simulink model "Sim_Riementrieb"  (R2015b)
settings: Solver=ode45  StartTime=0.0  StopTime=12  MaxStep=1e-3  RelTol=1e-7  AbsTol=1e-7
InitFcn:
  | set_parameter
undefined symbols (not defined in the file or in its folder): parRegid, parRegomegam, parSys
libraries: cstblocks x2
settings Model: Creator=wke  LastModifiedBy=jens
settings SolverCC: ShapePreserveControl=EnableAll
settings DataIOCC: SaveFormat=Array  SignalLoggingSaveFormat=ModelDataLogs
settings OptimizationCC: ExpressionDepthLimit=2147483647
settings DebuggingCC: UnderspecifiedInitializationDetection=Classic  MergeDetectMultiDrivingBlocksExec=none  SolverPrmCheckMsg=warning  FcnCallInpInsideContextMsg=UseLocalSettings  StateNameClashWarn=warning
settings HardwareCC: ProdBitPerPointer=32  ProdLargestAtomicFloat=None  ProdIntDivRoundTo=Undefined  ProdEndianess=Unspecified  ProdWordSize=32  ProdHWDeviceType=32-bit Generic
settings SFSimCC: SimParseCustomCode=off
settings GRTTargetCC: GeneratePreprocessorConditionals=Disable all  CombineOutputUpdateFcns=off  GRTInterface=on
settings ConfigComp: CovModelRefEnable=Off

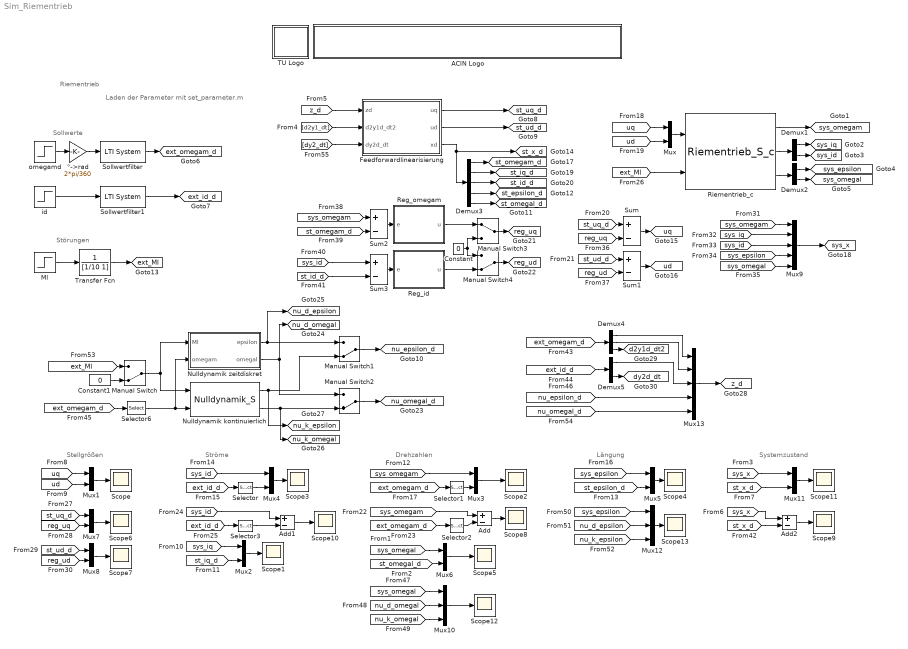
== system Sim_Riementrieb ==
  note: Riementrieb
  note: Laden der Parameter mit set_parameter.m
  note: Sollwerte
  note: Stellgrößen
  note: Ströme
  note: Drehzahlen
  note: Längung
  note: Störungen
  note: Systemzustand
  ACIN Logo : Subsystem
      mask init:
      | s = get_param(gcb,'UserData');
      mask Display:
      | image(s.logo,[0 0 439 45]);
      | %axis image
  Add : Sum  Inputs=+-
  Add1 : Sum  Inputs=+-
  Add2 : Sum  Inputs=+-
  Constant : Constant  Value=0
  Constant1 : Constant  Value=0
  Demux1 : Demux  Outputs=2
  Demux2 : Demux  Outputs=2
  Demux3 : Demux  Outputs=5
  Demux4 : Demux  Outputs=3
  Demux5 : Demux  Outputs=2
  Feedforwardlinearisierung : MATLAB Function  TreatAsAtomicUnit=on
  Manual Switch{,1..2,4} (4 alike) : ManualSwitch  CurrentSetting=0
  Manual Switch3 : ManualSwitch
  Ml : Step  Time=8  After=0.1  SampleTime=0
  Mux{,1..8,11} (10 alike) : Mux  Inputs=2
  Mux10 : Mux  Inputs=3
  Mux12 : Mux  Inputs=3
  Mux13 : Mux  Inputs=5
  Mux9 : Mux  Inputs=5
  Nulldynamik kontinuierlich : M-S-Function  FunctionName=Nulldynamik_S  Parameters=parSys
  Nulldynamik zeitdiskret : MATLAB Function  TreatAsAtomicUnit=on
  Reg_id : MATLAB Function  TreatAsAtomicUnit=on
  Reg_omegam : MATLAB Function  TreatAsAtomicUnit=on
  Riementrieb_c : S-Function  FunctionName=Riementrieb_S_c  Parameters=parSys  SFunctionDeploymentMode=off  EnableBusSupport=off
      mask Display:
      | port_label('input',1,'uq,ud');
      | port_label('input',2,'Ml');
      | port_label('output',1,'omegam');
      | port_label('output',2,'iq,id');
      | port_label('output',3,'epsilon,omegal');
  Scope{,1..13} (14 alike) : Scope
  Selector : Selector  InputPortWidth=2  IndexOptions=Index vector (dialog)  Indices=[1]  OutputSizes=1
  Selector1 : Selector  InputPortWidth=3  IndexOptions=Index vector (dialog)  Indices=[1]  OutputSizes=1
  Selector2 : Selector  InputPortWidth=3  IndexOptions=Index vector (dialog)  Indices=[1]  OutputSizes=1
  Selector3 : Selector  InputPortWidth=2  IndexOptions=Index vector (dialog)  Indices=[1]  OutputSizes=1
  Selector6 : Selector  InputPortWidth=3  IndexOptions=Index vector (dialog)  Indices=[1]  OutputSizes=1
  Sollwertfilter : cstblocks/LTI System  sys=parReg.ssSF  IC=[]
  Sollwertfilter1 : cstblocks/LTI System  sys=parReg.ssSFi  IC=[]
  Sum{,1..3} (4 alike) : Sum  Inputs=+-
  TU Logo : Subsystem
      mask init:
      | s = get_param(gcb,'UserData');
      mask Display: image(s.logo,[0 0 45 45]);
  Transfer Fcn : TransferFcn  Denominator=[1/10 1]
  id : Step  After=0.1  SampleTime=0
  omegamd : Step  Time=4  After=1000/60*360  SampleTime=0
  °->rad : Gain  Gain=2*pi/360
  tag scope: d2y1d_dt2=global, dy2d_dt=global, ext_Ml=global, ext_id_d=global, ext_omegam_d=global, nu_d_epsilon=global, nu_d_omegal=global, nu_epsilon_d=global, nu_k_epsilon=global, nu_k_omegal=global, nu_omegal_d=global, reg_ud=global, reg_uq=global, st_epsilon_d=global, st_id_d=global, st_iq_d=global, st_omegal_d=global, st_omegam_d=global, st_ud_d=global, st_uq_d=global, st_x_d=global, sys_epsilon=global, sys_id=global, sys_iq=global, sys_omegal=global, sys_omegam=global, sys_x=global, ud=global, uq=global, z_d=global
  wires:
  Mux/1 -> Riementrieb_c/1
  °->rad/1 -> Sollwertfilter/1
  Sollwertfilter/1 -> [ext_omegam_d]
  Demux1/1 -> [sys_iq]
  Demux1/2 -> [sys_id]
  Demux2/1 -> [sys_epsilon]
  Demux2/2 -> [sys_omegal]
  Sollwertfilter1/1 -> [ext_id_d]
  id/1 -> Sollwertfilter1/1
  [uq] -> Mux1/1
  [ud] -> Mux1/2
  Mux1/1 -> Scope/1
  [sys_iq] -> Mux2/1
  [st_iq_d] -> Mux2/2
  Mux2/1 -> Scope1/1
  [sys_omegam] -> Mux3/1
  Mux3/1 -> Scope2/1
  [sys_id] -> Mux4/1
  [ext_id_d] -> Selector/1
  Mux4/1 -> Scope3/1
  [sys_epsilon] -> Mux5/1
  Mux5/1 -> Scope4/1
  [sys_omegal] -> Mux6/1
  Mux6/1 -> Scope5/1
  [ext_omegam_d] -> Selector1/1
  Selector1/1 -> Mux3/2
  Selector/1 -> Mux4/2
  [st_epsilon_d] -> Mux5/2
  [st_omegal_d] -> Mux6/2
  Add/1 -> Scope8/1
  [sys_omegam] -> Add/1
  [ext_omegam_d] -> Selector2/1
  Selector2/1 -> Add/2
  Add1/1 -> Scope10/1
  [sys_id] -> Add1/1
  [ext_id_d] -> Selector3/1
  Selector3/1 -> Add1/2
  Ml/1 -> Transfer Fcn/1
  omegamd/1 -> °->rad/1
  Transfer Fcn/1 -> [ext_Ml]
  [ext_Ml] -> Riementrieb_c/2
  [st_uq_d] -> Mux7/1
  [reg_uq] -> Mux7/2
  Mux7/1 -> Scope6/1
  [st_ud_d] -> Mux8/1
  [reg_ud] -> Mux8/2
  Mux8/1 -> Scope7/1
  Riementrieb_c/2 -> Demux1/1
  Riementrieb_c/3 -> Demux2/1
  Riementrieb_c/1 -> [sys_omegam]
  [sys_omegam] -> Mux9/1
  [sys_iq] -> Mux9/2
  [sys_id] -> Mux9/3
  [sys_epsilon] -> Mux9/4
  [sys_omegal] -> Mux9/5
  Mux9/1 -> [sys_x]
  Mux11/1 -> Scope11/1
  [sys_x] -> Mux11/1
  [st_x_d] -> Mux11/2
  [uq] -> Mux/1
  [ud] -> Mux/2
  Demux3/4 -> [st_epsilon_d]
  Demux3/5 -> [st_omegal_d]
  Demux3/1 -> [st_omegam_d]
  Demux3/2 -> [st_iq_d]
  Demux3/3 -> [st_id_d]
  Add2/1 -> Scope9/1
  [sys_x] -> Add2/1
  [st_x_d] -> Add2/2
  [z_d] -> Feedforwardlinearisierung/1(zd)
  Feedforwardlinearisierung/1(uq) -> [st_uq_d]
  Feedforwardlinearisierung/2(ud) -> [st_ud_d]
  Feedforwardlinearisierung/3(xd) -> Demux3/1, [st_x_d]
  Nulldynamik zeitdiskret/1(epsilon) -> [nu_d_epsilon], Manual Switch1/1
  Nulldynamik zeitdiskret/2(omegal) -> [nu_d_omegal], Manual Switch2/1
  Nulldynamik kontinuierlich/1 -> [nu_k_epsilon], Manual Switch1/2
  Nulldynamik kontinuierlich/2 -> [nu_k_omegal], Manual Switch2/2
  [sys_omegal] -> Mux10/1
  [nu_d_omegal] -> Mux10/2
  [nu_k_omegal] -> Mux10/3
  Mux10/1 -> Scope12/1
  [ext_omegam_d] -> Selector6/1
  Selector6/1 -> Nulldynamik zeitdiskret/2(omegam), Nulldynamik kontinuierlich/2
  [sys_epsilon] -> Mux12/1
  [nu_d_epsilon] -> Mux12/2
  [nu_k_epsilon] -> Mux12/3
  Mux12/1 -> Scope13/1
  [ext_Ml] -> Manual Switch/1
  Constant1/1 -> Manual Switch/2
  Manual Switch/1 -> Nulldynamik zeitdiskret/1(Ml), Nulldynamik kontinuierlich/1
  Manual Switch1/1 -> [nu_epsilon_d]
  Manual Switch2/1 -> [nu_omegal_d]
  Mux13/1 -> [z_d]
  [ext_omegam_d] -> Demux4/1
  Demux4/1 -> Mux13/1
  Demux4/2 -> Mux13/2
  [ext_id_d] -> Demux5/1
  Demux5/1 -> Mux13/3
  [nu_omegal_d] -> Mux13/5
  [nu_epsilon_d] -> Mux13/4
  Demux4/3 -> [d2y1d_dt2]
  Demux5/2 -> [dy2d_dt]
  [d2y1_dt] -> Feedforwardlinearisierung/2(d2y1d_dt2)
  [dy2_dt] -> Feedforwardlinearisierung/3(dy2d_dt)
  Sum/1 -> [uq]
  [reg_uq] -> Sum/2
  [st_uq_d] -> Sum/1
  Sum1/1 -> [ud]
  [st_ud_d] -> Sum1/1
  [reg_ud] -> Sum1/2
  Manual Switch3/1 -> [reg_uq]
  Manual Switch4/1 -> [reg_ud]
  Constant/1 -> Manual Switch3/2, Manual Switch4/1
  Reg_id/1(u) -> Manual Switch4/2
  Reg_omegam/1(u) -> Manual Switch3/1
  [sys_omegam] -> Sum2/1
  [st_omegam_d] -> Sum2/2
  Sum3/1 -> Reg_id/1(e)
  Sum2/1 -> Reg_omegam/1(e)
  [sys_id] -> Sum3/1
  [st_id_d] -> Sum3/2

== system Sim_Riementrieb/ACIN Logo ==

== system Sim_Riementrieb/TU Logo ==

== matlab function Sim_Riementrieb/Nulldynamik zeitdiskret ==
  settings: updateMethod=DISCRETE  sampleTime=parSys.TsID
  data: Ml input; omegam input; epsilon output; parSys parameter; omegal output
function [epsilon, omegal] = fcn(Ml,omegam,parSys)
%#codegen

persistent etakm1;
persistent ukm1;

if isempty(etakm1) || isempty(ukm1)
    etakm1  = [parSys.eta_1_0 parSys.eta_2_0];
    ukm1    = [Ml omegam];
    epsilon = etakm1(1);
    omegal  = etakm1(2);
    return;
end

Il  = parSys.Il;
cr1 = parSys.cr1;
cr3 = parSys.cr3;
dl  = parSys.dl;
rl  = parSys.rl;
Im  = parSys.Im;
dm  = parSys.dm;
rm  = parSys.rm;
Rm  = parSys.Rm;
Lm  = parSys.Lm;
p   = parSys.p;
Phi = parSys.Phi;

Mlk     = Ml;
omegamk = omegam;

epsilon = etakm1(1);
omegal  = etakm1(2);
Ml      = ukm1(1);
omegam  = ukm1(2);

etapkm1 = [omegal * rl - omegam * rm 1 / Il * (-2 * (cr3 * epsilon ^ 3 + cr1 * epsilon) * rl - dl * omegal + Ml)];

etakP = etakm1 + parSys.TsID * etapkm1;

epsilon = etakP(1);
omegal  = etakP(2);
Ml     = Mlk;
omegam = omegamk;

etapP = [omegal * rl - omegam * rm 1 / Il * (-2 * (cr3 * epsilon ^ 3 + cr1 * epsilon) * rl - dl * omegal + Ml)];

etak = etakm1 + parSys.TsID / 2 * (etapkm1 + etapP);

epsilon = etak(1);
omegal  = etak(2);

etakm1 = etak;
ukm1 = [Mlk omegamk];

== matlab function Sim_Riementrieb/Feedforwardlinearisierung ==
  data: zd input; d2y1d_dt2 input; dy2d_dt input; uq output; parSys parameter; ud output; xd output size=5
function [uq, ud, xd] = fcn(zd, d2y1d_dt2, dy2d_dt, parSys)
%#codegen

Il  = parSys.Il;
cr1 = parSys.cr1;
cr3 = parSys.cr3;
dl  = parSys.dl;
rl  = parSys.rl;
I_m  = parSys.Im;
dm  = parSys.dm;
rm  = parSys.rm;
Rm  = parSys.Rm;
Lm  = parSys.Lm;
p   = parSys.p;
Phi = parSys.Phi;

%Muss noch geändert werden
z1 = zd(1);
z2 = zd(2);
z3 = zd(3);
z4 = zd(4);
z5 = zd(5);

omegam = z1;
iq = 0.2e1 / 0.3e1 * (-2 * cr3 * rm * z4 ^ 3 - 2 * cr1 * rm * z4 + z2 * I_m + dm * z1) / p / Phi;
id = z3;
epsilon = z4; 
omegal = z5;

Lg1h1 = [0];
Lg2h1 = [0];
Lfh1 = [0.1e1 / I_m * ((2 * (cr3 * epsilon ^ 3 + cr1 * epsilon) * rm) - dm * omegam + 0.3e1 / 0.2e1 * p * Phi * iq)];
Lg1Lfh1 = [0.1e1 / I_m * p * Phi / Lm];
Lg2Lfh1 = [0];
Lf2h1 = [-0.1e1 / I_m ^ 2 * dm * ((2 * (cr3 * epsilon ^ 3 + cr1 * epsilon) * rm) - dm * omegam + 0.3e1 / 0.2e1 * p * Phi * iq) + 0.1e1 / I_m * p * Phi / Lm * (-Rm * iq + 0.3e1 / 0.2e1 * Lm * p * omegam * id - Phi * p * omegam) + 0.2e1 / I_m * (3 * cr3 * epsilon ^ 2 + cr1) * rm * (omegal * rl - omegam * rm)];
Lfh2 = [0.2e1 / 0.3e1 / Lm * (-Rm * id - 0.3e1 / 0.2e1 * Lm * p * omegam * iq)];
Lg1h2 = [0];
Lg2h2 = [0.2e1 / 0.3e1 / Lm];
vv = [d2y1d_dt2; dy2d_dt];
bb = [Lf2h1; Lfh2];
DD_inv = [Lg2h2 / (Lg1Lfh1 * Lg2h2 - Lg1h2 * Lg2Lfh1) -Lg2Lfh1 / (Lg1Lfh1 * Lg2h2 - Lg1h2 * Lg2Lfh1); -Lg1h2 / (Lg1Lfh1 * Lg2h2 - Lg1h2 * Lg2Lfh1) Lg1Lfh1 / (Lg1Lfh1 * Lg2h2 - Lg1h2 * Lg2Lfh1);];
u = DD_inv * (vv - bb);


uq = u(1);
ud = u(2);

xd = [omegam; iq; id; epsilon; omegal];

== matlab function Sim_Riementrieb/Reg_omegam ==
  settings: updateMethod=DISCRETE  sampleTime=parSys.TsID
  data: u output; e input; parRegomegam parameter; parSys parameter
function u = Reg_omegam(e, parRegomegam, parSys)
%#codegen

persistent eI;
if isempty(eI)
    eI = 0;
end

u = parRegomegam.Kp * e + parRegomegam.Ki * eI;

eI = eI + parSys.TsID * e;

== matlab function Sim_Riementrieb/Reg_id ==
  settings: updateMethod=DISCRETE  sampleTime=parSys.TsID
  data: u output; e input; parRegid parameter; parSys parameter
function u = Reg_id(e, parRegid, parSys)
%#codegen

persistent eI;
if isempty(eI)
    eI = 0;
end

u = parRegid.Kp * e + parRegid.Ki * eI;

eI = eI + parSys.TsID * e;
